simulink model "RobotX_ss_acousticsSKIP_dock_odoa_ta_1021"  (R2014a)
settings: Solver=FixedStepDiscrete  StartTime=0.0  StopTime=inf  FixedStep=.25  RelTol=1e-3
undefined symbols (not defined in the file): Com1, Com2, Com3, Com4, DiscIntNeverNeededParam, standard
libraries: xpcseriallib x42, simulink x8, slrtlib x8, speedgoatlib x2, speedgoatlib_IO102 x1
(part 5 of 19)

== matlab function RobotX_ss_acousticsSKIP_dock_odoa_ta_1021/Main FSM/ODOA/SLAM1/Models for prediction/Model10/Dynamic Model ==
  data: F_surge input; F_sway input; Torque input; u input; surgeAccel output; v input; psi input; swayAccel output; yawAccel output
function [surgeAccel, swayAccel, yawAccel] = ...
    WAM_V_3DOF(F_surge, F_sway, Torque, u, v, psi)
%Written by Anderson Lebbad on August 12, 2014
%Last Edited:

%This function was heavily based off of Ariel Qu's Vel3DOF_IvanV1. It was
%rewritten for real-time use.

%This function will produce the transient output surge velocity of a
%linearized model of the USV. It is assumed that the vehicle is equivalent
%to two cylinders in the water.

%%%%%DEFINED VARIABLE%%%%%%
%
%   Xext = Thrust from motors
%   Next = Moment from motor
%   m = Mass of vehicle
%   Xudot = Added mass in surge direction
%   Yvdot = Added mass in sway direction
%   Nrdot = Added mass from yaw
%   xg = offset from center of gravity
%   rho = density of seawater
%   S = wetted surface area
%   R = Reynolds number
%   Cd = Coefficient of drag
%   Cdc = Coefficient of drag for sway
%   nu = Kinematic viscosity
%   L = Length overall
%   T = draft
%   B = beam
%   SA = Surface area of cylinder experiencing sway
%   Iz = moment of inertia about Z axis
%
%%%%%%

% Force/Mometns from thrusters & control surfaces...

tau = [F_surge; F_sway; Torque];

% Calculate yaw rate
persistent lastHeading
if isempty(lastHeading)
    lastHeading = psi;
end
%Sample time
ts = .1;

r = (psi - lastHeading)/ts;

% Velocity & Angular velocity vectors
vel = [u; v; 0];
omega = [0; 0; r];

%define variables
m = 145.7;         % Total mass [kg] - reduced from 102
rho = 1025.9;   % density of seawater [kg/m^3]
L = 3.91*0.85;  % Length on the waterline [m]
B = 0.426;       % Demihull beam [m]
T = B*0.2;        % Draft of the demihull [m]
p_bar = 1.0; % sidehull separation - from centerplane vessel to centerplane demihull
Iz = 262.181;    % Mass moment of inertia about z-axis [kg*m^2]
xg = 0;         % Body-Fixed coordinate system taken to be center of gravity
yg = 0;         % Symmetrical Vessel
Cd = 1.1;       % Drag coefficient for a lateral cylinder
LCG = 1.485;        % Need to know where LCG wrt stern

% Vector location of port and starboard hulls
r_port = [-LCG; -p_bar; 0];   
r_stbd = [-LCG; p_bar; 0];

% Port and starboard hull velocities
vel_port = vel + cross(omega,r_port);
vel_stbd = vel + cross(omega,r_stbd);

u_port = vel_port(1);
u_stbd = vel_stbd(1);

% Port and starboard state vectors
state_port = vel_port + omega;
state_stbd = vel_stbd + omega;

%% Added Mass
% Estimated for each hull, then multiplied by 2 to account for both hulls
Xudot = -0.05*m;

%Using strip theory to estimate added mass coefficients
Nrdot = -(4.75/2*pi*rho*p_bar*T^4 + pi*rho*T^2*((L - LCG)^3 + LCG^3)/3);
Nvdot = - pi*rho*T^2*((L - LCG)^2 - LCG^2)/2;

Yrdot = Nvdot;
Yvdot = -rho*pi*T^2*L;

% Multiply by 2:
Xudot = 2*Xudot;
Nrdot = 2*Nrdot;
Nvdot = 2*Nvdot;
Yrdot = 2*Yrdot;
Yvdot = 2*Yvdot;

%Calculate Coefficient of Drag for Sway from 1950 SNAME approximation
Cdc= 1.1 + 0.0045*L/T - 0.1*B/T + 0.016*(B/T)^2;
SA = 2*pi/4*T*L; %projected area of pontoon for two pontoons

%% Linear Drag Terms
%Total Speed
U = sqrt(u^2+v^2);

Xu = 0;
Yv = -0.5*rho*abs(v)*2*Cdc*SA; %20 was the last working number %from SNAME 1950, x2 for two cylinders
%Nr = -0.5*pi*rho*U*T^2*L^2;
Nr = -pi*rho*U*T^2*L^2*.065;
Nv = -pi*rho*U*T^2*L*.01;
Yr = pi*rho*U*T^2*L*0.2;  %from Newman approximation in Lewandowski

%% Nonlinear Drag Terms

% Drag and Moment due to drag on entire vessel - includes nonlinear and
% linear drag terms
D_port = 0.5*(0.44*u_port^3 - 0.01*u_port^2 + 19*u_port);     % Can assume that this equation also takes into account Xu - so set Xu=0
D_stbd = 0.5*(0.44*u_stbd^3 - 0.01*u_stbd^2 + 19*u_stbd);     % Can assume that this equation also takes into account Xu - so set Xu=0

tau_drag = [-(D_port + D_stbd); 0; (D_stbd - D_port)*p_bar];

Xuu = 0;

%% Maneuvering Coefficient Matrices
% Added Mass Matrix
M = [(m - Xudot)      0              0;...
    0               (m - Yvdot)     (m*xg - Yrdot);...
    0               (m*xg - Nvdot)  (Iz - Nrdot)];

%Centripetal and Added Mass Centripetal force matrices
% C_RB = [
%     0                  0                0
%     0                  0                0
%     0                  0                0
%     ];

% C_RB = [
%     0                  0                -m*(xg*r + v)
%     0                  0                -m*(yg*r - u)
%     m*(xg*r + v)       m*(yg*r - u)     0
%     ];

% C_A = -[ %negative originally
%     0                               0           0
%     0                               0           0
%     0                               0           0
%     ];

% Negating centripetal acceleration for test
C_RB = 0;
C_A = 0;

D = -[Xu  0   0;...
      0   Yv  Yr;...
      0   Nv  Nr];

% Nonlinear Drag Coefficients
D_N = -[Xuu*u   0                       0;...
        0       0                       0;...
        0       0                       0];
    
%% Calculate the port and starboard force vectors
tau_port = -(C_RB + C_A + D + D_N)*state_port;
tau_stbd = -(C_RB + C_A + D + D_N)*state_stbd;


%% Sum the force vectors
tau_tot = tau + tau_drag + tau_port + tau_stbd...
    + cross(r_port,[tau_port(1);tau_port(2);0]) + ...
    cross(r_stbd,[tau_stbd(1);tau_stbd(2);0]);

% Calculate the time derivative of the state vector

accel = M\tau_tot;

%% Separate output

surgeAccel = accel(1);
swayAccel = accel(2);
yawAccel = accel(3);

end

== matlab function RobotX_ss_acousticsSKIP_dock_odoa_ta_1021/Main FSM/ODOA/SLAM1/Models for prediction/Model13/Stbd Thruster Model ==
  data: stbdMP input; F_surge output; stbdAzimuth input; F_sway output; Torque output
function [F_surge,F_sway,Torque]  = StarBoardThruster(stbdMP,stbdAzimuth)
%Approximation for Starboard Force and Moment with the input motor power
%and azimuth angle of thruster

%Longitudinal distance from center of mass
longDist =1.007;           %m

%Axial distance from center of mass
axialDist=1.485;            %m

%% Piece-wise thrust calculation

if stbdMP <= -51.0119
    F = .9140*stbdMP + 40;
elseif stbdMP >= 26.8367
    F = 1.658*stbdMP - 41.01;
else
    F = .12987*stbdMP;
end

%% Force components
F_surge=F*cos(stbdAzimuth*pi/180);       %N
F_sway=F*sin(stbdAzimuth*pi/180);       %N

%% Torque calculation

Torque = -F_surge*longDist - F_sway*axialDist;   %N.m

end

== matlab function RobotX_ss_acousticsSKIP_dock_odoa_ta_1021/Main FSM/ODOA/SLAM1/Models for prediction/Model14/Dynamic Model ==
  data: F_surge input; F_sway input; Torque input; u input; surgeAccel output; v input; psi input; swayAccel output; yawAccel output
function [surgeAccel, swayAccel, yawAccel] = ...
    WAM_V_3DOF(F_surge, F_sway, Torque, u, v, psi)
%Written by Anderson Lebbad on August 12, 2014
%Last Edited:

%This function was heavily based off of Ariel Qu's Vel3DOF_IvanV1. It was
%rewritten for real-time use.

%This function will produce the transient output surge velocity of a
%linearized model of the USV. It is assumed that the vehicle is equivalent
%to two cylinders in the water.

%%%%%DEFINED VARIABLE%%%%%%
%
%   Xext = Thrust from motors
%   Next = Moment from motor
%   m = Mass of vehicle
%   Xudot = Added mass in surge direction
%   Yvdot = Added mass in sway direction
%   Nrdot = Added mass from yaw
%   xg = offset from center of gravity
%   rho = density of seawater
%   S = wetted surface area
%   R = Reynolds number
%   Cd = Coefficient of drag
%   Cdc = Coefficient of drag for sway
%   nu = Kinematic viscosity
%   L = Length overall
%   T = draft
%   B = beam
%   SA = Surface area of cylinder experiencing sway
%   Iz = moment of inertia about Z axis
%
%%%%%%

% Force/Mometns from thrusters & control surfaces...

tau = [F_surge; F_sway; Torque];

% Calculate yaw rate
persistent lastHeading
if isempty(lastHeading)
    lastHeading = psi;
end
%Sample time
ts = .1;

r = (psi - lastHeading)/ts;

% Velocity & Angular velocity vectors
vel = [u; v; 0];
omega = [0; 0; r];

%define variables
m = 145.7;         % Total mass [kg] - reduced from 102
rho = 1025.9;   % density of seawater [kg/m^3]
L = 3.91*0.85;  % Length on the waterline [m]
B = 0.426;       % Demihull beam [m]
T = B*0.2;        % Draft of the demihull [m]
p_bar = 1.0; % sidehull separation - from centerplane vessel to centerplane demihull
Iz = 262.181;    % Mass moment of inertia about z-axis [kg*m^2]
xg = 0;         % Body-Fixed coordinate system taken to be center of gravity
yg = 0;         % Symmetrical Vessel
Cd = 1.1;       % Drag coefficient for a lateral cylinder
LCG = 1.485;        % Need to know where LCG wrt stern

% Vector location of port and starboard hulls
r_port = [-LCG; -p_bar; 0];   
r_stbd = [-LCG; p_bar; 0];

% Port and starboard hull velocities
vel_port = vel + cross(omega,r_port);
vel_stbd = vel + cross(omega,r_stbd);

u_port = vel_port(1);
u_stbd = vel_stbd(1);

% Port and starboard state vectors
state_port = vel_port + omega;
state_stbd = vel_stbd + omega;

%% Added Mass
% Estimated for each hull, then multiplied by 2 to account for both hulls
Xudot = -0.05*m;

%Using strip theory to estimate added mass coefficients
Nrdot = -(4.75/2*pi*rho*p_bar*T^4 + pi*rho*T^2*((L - LCG)^3 + LCG^3)/3);
Nvdot = - pi*rho*T^2*((L - LCG)^2 - LCG^2)/2;

Yrdot = Nvdot;
Yvdot = -rho*pi*T^2*L;

% Multiply by 2:
Xudot = 2*Xudot;
Nrdot = 2*Nrdot;
Nvdot = 2*Nvdot;
Yrdot = 2*Yrdot;
Yvdot = 2*Yvdot;

%Calculate Coefficient of Drag for Sway from 1950 SNAME approximation
Cdc= 1.1 + 0.0045*L/T - 0.1*B/T + 0.016*(B/T)^2;
SA = 2*pi/4*T*L; %projected area of pontoon for two pontoons

%% Linear Drag Terms
%Total Speed
U = sqrt(u^2+v^2);

Xu = 0;
Yv = -0.5*rho*abs(v)*2*Cdc*SA; %20 was the last working number %from SNAME 1950, x2 for two cylinders
%Nr = -0.5*pi*rho*U*T^2*L^2;
Nr = -pi*rho*U*T^2*L^2*.065;
Nv = -pi*rho*U*T^2*L*.01;
Yr = pi*rho*U*T^2*L*0.2;  %from Newman approximation in Lewandowski

%% Nonlinear Drag Terms

% Drag and Moment due to drag on entire vessel - includes nonlinear and
% linear drag terms
D_port = 0.5*(0.44*u_port^3 - 0.01*u_port^2 + 19*u_port);     % Can assume that this equation also takes into account Xu - so set Xu=0
D_stbd = 0.5*(0.44*u_stbd^3 - 0.01*u_stbd^2 + 19*u_stbd);     % Can assume that this equation also takes into account Xu - so set Xu=0

tau_drag = [-(D_port + D_stbd); 0; (D_stbd - D_port)*p_bar];

Xuu = 0;

%% Maneuvering Coefficient Matrices
% Added Mass Matrix
M = [(m - Xudot)      0              0;...
    0               (m - Yvdot)     (m*xg - Yrdot);...
    0               (m*xg - Nvdot)  (Iz - Nrdot)];

%Centripetal and Added Mass Centripetal force matrices
% C_RB = [
%     0                  0                0
%     0                  0                0
%     0                  0                0
%     ];

% C_RB = [
%     0                  0                -m*(xg*r + v)
%     0                  0                -m*(yg*r - u)
%     m*(xg*r + v)       m*(yg*r - u)     0
%     ];

% C_A = -[ %negative originally
%     0                               0           0
%     0                               0           0
%     0                               0           0
%     ];

% Negating centripetal acceleration for test
C_RB = 0;
C_A = 0;

D = -[Xu  0   0;...
      0   Yv  Yr;...
      0   Nv  Nr];

% Nonlinear Drag Coefficients
D_N = -[Xuu*u   0                       0;...
        0       0                       0;...
        0       0                       0];
    
%% Calculate the port and starboard force vectors
tau_port = -(C_RB + C_A + D + D_N)*state_port;
tau_stbd = -(C_RB + C_A + D + D_N)*state_stbd;


%% Sum the force vectors
tau_tot = tau + tau_drag + tau_port + tau_stbd...
    + cross(r_port,[tau_port(1);tau_port(2);0]) + ...
    cross(r_stbd,[tau_stbd(1);tau_stbd(2);0]);

% Calculate the time derivative of the state vector

accel = M\tau_tot;

%% Separate output

surgeAccel = accel(1);
swayAccel = accel(2);
yawAccel = accel(3);

end

== matlab function RobotX_ss_acousticsSKIP_dock_odoa_ta_1021/Main FSM/ODOA/SLAM1/Models for prediction/Model17/Stbd Thruster Model ==
  data: stbdMP input; F_surge output; stbdAzimuth input; F_sway output; Torque output
function [F_surge,F_sway,Torque]  = StarBoardThruster(stbdMP,stbdAzimuth)
%Approximation for Starboard Force and Moment with the input motor power
%and azimuth angle of thruster

%Longitudinal distance from center of mass
longDist =1.007;           %m

%Axial distance from center of mass
axialDist=1.485;            %m

%% Piece-wise thrust calculation

if stbdMP <= -51.0119
    F = .9140*stbdMP + 40;
elseif stbdMP >= 26.8367
    F = 1.658*stbdMP - 41.01;
else
    F = .12987*stbdMP;
end

%% Force components
F_surge=F*cos(stbdAzimuth*pi/180);       %N
F_sway=F*sin(stbdAzimuth*pi/180);       %N

%% Torque calculation

Torque = -F_surge*longDist - F_sway*axialDist;   %N.m

end

== matlab function RobotX_ss_acousticsSKIP_dock_odoa_ta_1021/Main FSM/ODOA/SLAM1/Models for prediction/Model18/Dynamic Model ==
  data: F_surge input; F_sway input; Torque input; u input; surgeAccel output; v input; psi input; swayAccel output; yawAccel output
function [surgeAccel, swayAccel, yawAccel] = ...
    WAM_V_3DOF(F_surge, F_sway, Torque, u, v, psi)
%Written by Anderson Lebbad on August 12, 2014
%Last Edited:

%This function was heavily based off of Ariel Qu's Vel3DOF_IvanV1. It was
%rewritten for real-time use.

%This function will produce the transient output surge velocity of a
%linearized model of the USV. It is assumed that the vehicle is equivalent
%to two cylinders in the water.

%%%%%DEFINED VARIABLE%%%%%%
%
%   Xext = Thrust from motors
%   Next = Moment from motor
%   m = Mass of vehicle
%   Xudot = Added mass in surge direction
%   Yvdot = Added mass in sway direction
%   Nrdot = Added mass from yaw
%   xg = offset from center of gravity
%   rho = density of seawater
%   S = wetted surface area
%   R = Reynolds number
%   Cd = Coefficient of drag
%   Cdc = Coefficient of drag for sway
%   nu = Kinematic viscosity
%   L = Length overall
%   T = draft
%   B = beam
%   SA = Surface area of cylinder experiencing sway
%   Iz = moment of inertia about Z axis
%
%%%%%%

% Force/Mometns from thrusters & control surfaces...

tau = [F_surge; F_sway; Torque];

% Calculate yaw rate
persistent lastHeading
if isempty(lastHeading)
    lastHeading = psi;
end
%Sample time
ts = .1;

r = (psi - lastHeading)/ts;

% Velocity & Angular velocity vectors
vel = [u; v; 0];
omega = [0; 0; r];

%define variables
m = 145.7;         % Total mass [kg] - reduced from 102
rho = 1025.9;   % density of seawater [kg/m^3]
L = 3.91*0.85;  % Length on the waterline [m]
B = 0.426;       % Demihull beam [m]
T = B*0.2;        % Draft of the demihull [m]
p_bar = 1.0; % sidehull separation - from centerplane vessel to centerplane demihull
Iz = 262.181;    % Mass moment of inertia about z-axis [kg*m^2]
xg = 0;         % Body-Fixed coordinate system taken to be center of gravity
yg = 0;         % Symmetrical Vessel
Cd = 1.1;       % Drag coefficient for a lateral cylinder
LCG = 1.485;        % Need to know where LCG wrt stern

% Vector location of port and starboard hulls
r_port = [-LCG; -p_bar; 0];   
r_stbd = [-LCG; p_bar; 0];

% Port and starboard hull velocities
vel_port = vel + cross(omega,r_port);
vel_stbd = vel + cross(omega,r_stbd);

u_port = vel_port(1);
u_stbd = vel_stbd(1);

% Port and starboard state vectors
state_port = vel_port + omega;
state_stbd = vel_stbd + omega;

%% Added Mass
% Estimated for each hull, then multiplied by 2 to account for both hulls
Xudot = -0.05*m;

%Using strip theory to estimate added mass coefficients
Nrdot = -(4.75/2*pi*rho*p_bar*T^4 + pi*rho*T^2*((L - LCG)^3 + LCG^3)/3);
Nvdot = - pi*rho*T^2*((L - LCG)^2 - LCG^2)/2;

Yrdot = Nvdot;
Yvdot = -rho*pi*T^2*L;

% Multiply by 2:
Xudot = 2*Xudot;
Nrdot = 2*Nrdot;
Nvdot = 2*Nvdot;
Yrdot = 2*Yrdot;
Yvdot = 2*Yvdot;

%Calculate Coefficient of Drag for Sway from 1950 SNAME approximation
Cdc= 1.1 + 0.0045*L/T - 0.1*B/T + 0.016*(B/T)^2;
SA = 2*pi/4*T*L; %projected area of pontoon for two pontoons

%% Linear Drag Terms
%Total Speed
U = sqrt(u^2+v^2);

Xu = 0;
Yv = -0.5*rho*abs(v)*2*Cdc*SA; %20 was the last working number %from SNAME 1950, x2 for two cylinders
%Nr = -0.5*pi*rho*U*T^2*L^2;
Nr = -pi*rho*U*T^2*L^2*.065;
Nv = -pi*rho*U*T^2*L*.01;
Yr = pi*rho*U*T^2*L*0.2;  %from Newman approximation in Lewandowski

%% Nonlinear Drag Terms

% Drag and Moment due to drag on entire vessel - includes nonlinear and
% linear drag terms
D_port = 0.5*(0.44*u_port^3 - 0.01*u_port^2 + 19*u_port);     % Can assume that this equation also takes into account Xu - so set Xu=0
D_stbd = 0.5*(0.44*u_stbd^3 - 0.01*u_stbd^2 + 19*u_stbd);     % Can assume that this equation also takes into account Xu - so set Xu=0

tau_drag = [-(D_port + D_stbd); 0; (D_stbd - D_port)*p_bar];

Xuu = 0;

%% Maneuvering Coefficient Matrices
% Added Mass Matrix
M = [(m - Xudot)      0              0;...
    0               (m - Yvdot)     (m*xg - Yrdot);...
    0               (m*xg - Nvdot)  (Iz - Nrdot)];

%Centripetal and Added Mass Centripetal force matrices
% C_RB = [
%     0                  0                0
%     0                  0                0
%     0                  0                0
%     ];

% C_RB = [
%     0                  0                -m*(xg*r + v)
%     0                  0                -m*(yg*r - u)
%     m*(xg*r + v)       m*(yg*r - u)     0
%     ];

% C_A = -[ %negative originally
%     0                               0           0
%     0                               0           0
%     0                               0           0
%     ];

% Negating centripetal acceleration for test
C_RB = 0;
C_A = 0;

D = -[Xu  0   0;...
      0   Yv  Yr;...
      0   Nv  Nr];

% Nonlinear Drag Coefficients
D_N = -[Xuu*u   0                       0;...
        0       0                       0;...
        0       0                       0];
    
%% Calculate the port and starboard force vectors
tau_port = -(C_RB + C_A + D + D_N)*state_port;
tau_stbd = -(C_RB + C_A + D + D_N)*state_stbd;


%% Sum the force vectors
tau_tot = tau + tau_drag + tau_port + tau_stbd...
    + cross(r_port,[tau_port(1);tau_port(2);0]) + ...
    cross(r_stbd,[tau_stbd(1);tau_stbd(2);0]);

% Calculate the time derivative of the state vector

accel = M\tau_tot;

%% Separate output

surgeAccel = accel(1);
swayAccel = accel(2);
yawAccel = accel(3);

end

== matlab function RobotX_ss_acousticsSKIP_dock_odoa_ta_1021/Main FSM/ODOA/SLAM1/Models for prediction/Model20/Stbd Thruster Model ==
  data: stbdMP input; F_surge output; stbdAzimuth input; F_sway output; Torque output
function [F_surge,F_sway,Torque]  = StarBoardThruster(stbdMP,stbdAzimuth)
%Approximation for Starboard Force and Moment with the input motor power
%and azimuth angle of thruster

%Longitudinal distance from center of mass
longDist =1.007;           %m

%Axial distance from center of mass
axialDist=1.485;            %m

%% Piece-wise thrust calculation

if stbdMP <= -51.0119
    F = .9140*stbdMP + 40;
elseif stbdMP >= 26.8367
    F = 1.658*stbdMP - 41.01;
else
    F = .12987*stbdMP;
end

%% Force components
F_surge=F*cos(stbdAzimuth*pi/180);       %N
F_sway=F*sin(stbdAzimuth*pi/180);       %N

%% Torque calculation

Torque = -F_surge*longDist - F_sway*axialDist;   %N.m

end

== matlab function RobotX_ss_acousticsSKIP_dock_odoa_ta_1021/Main FSM/ODOA/SLAM1/Models for prediction/Model21/Dynamic Model ==
  data: F_surge input; F_sway input; Torque input; u input; surgeAccel output; v input; psi input; swayAccel output; yawAccel output
function [surgeAccel, swayAccel, yawAccel] = ...
    WAM_V_3DOF(F_surge, F_sway, Torque, u, v, psi)
%Written by Anderson Lebbad on August 12, 2014
%Last Edited:

%This function was heavily based off of Ariel Qu's Vel3DOF_IvanV1. It was
%rewritten for real-time use.

%This function will produce the transient output surge velocity of a
%linearized model of the USV. It is assumed that the vehicle is equivalent
%to two cylinders in the water.

%%%%%DEFINED VARIABLE%%%%%%
%
%   Xext = Thrust from motors
%   Next = Moment from motor
%   m = Mass of vehicle
%   Xudot = Added mass in surge direction
%   Yvdot = Added mass in sway direction
%   Nrdot = Added mass from yaw
%   xg = offset from center of gravity
%   rho = density of seawater
%   S = wetted surface area
%   R = Reynolds number
%   Cd = Coefficient of drag
%   Cdc = Coefficient of drag for sway
%   nu = Kinematic viscosity
%   L = Length overall
%   T = draft
%   B = beam
%   SA = Surface area of cylinder experiencing sway
%   Iz = moment of inertia about Z axis
%
%%%%%%

% Force/Mometns from thrusters & control surfaces...

tau = [F_surge; F_sway; Torque];

% Calculate yaw rate
persistent lastHeading
if isempty(lastHeading)
    lastHeading = psi;
end
%Sample time
ts = .1;

r = (psi - lastHeading)/ts;

% Velocity & Angular velocity vectors
vel = [u; v; 0];
omega = [0; 0; r];

%define variables
m = 145.7;         % Total mass [kg] - reduced from 102
rho = 1025.9;   % density of seawater [kg/m^3]
L = 3.91*0.85;  % Length on the waterline [m]
B = 0.426;       % Demihull beam [m]
T = B*0.2;        % Draft of the demihull [m]
p_bar = 1.0; % sidehull separation - from centerplane vessel to centerplane demihull
Iz = 262.181;    % Mass moment of inertia about z-axis [kg*m^2]
xg = 0;         % Body-Fixed coordinate system taken to be center of gravity
yg = 0;         % Symmetrical Vessel
Cd = 1.1;       % Drag coefficient for a lateral cylinder
LCG = 1.485;        % Need to know where LCG wrt stern

% Vector location of port and starboard hulls
r_port = [-LCG; -p_bar; 0];   
r_stbd = [-LCG; p_bar; 0];

% Port and starboard hull velocities
vel_port = vel + cross(omega,r_port);
vel_stbd = vel + cross(omega,r_stbd);

u_port = vel_port(1);
u_stbd = vel_stbd(1);

% Port and starboard state vectors
state_port = vel_port + omega;
state_stbd = vel_stbd + omega;

%% Added Mass
% Estimated for each hull, then multiplied by 2 to account for both hulls
Xudot = -0.05*m;

%Using strip theory to estimate added mass coefficients
Nrdot = -(4.75/2*pi*rho*p_bar*T^4 + pi*rho*T^2*((L - LCG)^3 + LCG^3)/3);
Nvdot = - pi*rho*T^2*((L - LCG)^2 - LCG^2)/2;

Yrdot = Nvdot;
Yvdot = -rho*pi*T^2*L;

% Multiply by 2:
Xudot = 2*Xudot;
Nrdot = 2*Nrdot;
Nvdot = 2*Nvdot;
Yrdot = 2*Yrdot;
Yvdot = 2*Yvdot;

%Calculate Coefficient of Drag for Sway from 1950 SNAME approximation
Cdc= 1.1 + 0.0045*L/T - 0.1*B/T + 0.016*(B/T)^2;
SA = 2*pi/4*T*L; %projected area of pontoon for two pontoons

%% Linear Drag Terms
%Total Speed
U = sqrt(u^2+v^2);

Xu = 0;
Yv = -0.5*rho*abs(v)*2*Cdc*SA; %20 was the last working number %from SNAME 1950, x2 for two cylinders
%Nr = -0.5*pi*rho*U*T^2*L^2;
Nr = -pi*rho*U*T^2*L^2*.065;
Nv = -pi*rho*U*T^2*L*.01;
Yr = pi*rho*U*T^2*L*0.2;  %from Newman approximation in Lewandowski

%% Nonlinear Drag Terms

% Drag and Moment due to drag on entire vessel - includes nonlinear and
% linear drag terms
D_port = 0.5*(0.44*u_port^3 - 0.01*u_port^2 + 19*u_port);     % Can assume that this equation also takes into account Xu - so set Xu=0
D_stbd = 0.5*(0.44*u_stbd^3 - 0.01*u_stbd^2 + 19*u_stbd);     % Can assume that this equation also takes into account Xu - so set Xu=0

tau_drag = [-(D_port + D_stbd); 0; (D_stbd - D_port)*p_bar];

Xuu = 0;

%% Maneuvering Coefficient Matrices
% Added Mass Matrix
M = [(m - Xudot)      0              0;...
    0               (m - Yvdot)     (m*xg - Yrdot);...
    0               (m*xg - Nvdot)  (Iz - Nrdot)];

%Centripetal and Added Mass Centripetal force matrices
% C_RB = [
%     0                  0                0
%     0                  0                0
%     0                  0                0
%     ];

% C_RB = [
%     0                  0                -m*(xg*r + v)
%     0                  0                -m*(yg*r - u)
%     m*(xg*r + v)       m*(yg*r - u)     0
%     ];

% C_A = -[ %negative originally
%     0                               0           0
%     0                               0           0
%     0                               0           0
%     ];

% Negating centripetal acceleration for test
C_RB = 0;
C_A = 0;

D = -[Xu  0   0;...
      0   Yv  Yr;...
      0   Nv  Nr];

% Nonlinear Drag Coefficients
D_N = -[Xuu*u   0                       0;...
        0       0                       0;...
        0       0                       0];
    
%% Calculate the port and starboard force vectors
tau_port = -(C_RB + C_A + D + D_N)*state_port;
tau_stbd = -(C_RB + C_A + D + D_N)*state_stbd;


%% Sum the force vectors
tau_tot = tau + tau_drag + tau_port + tau_stbd...
    + cross(r_port,[tau_port(1);tau_port(2);0]) + ...
    cross(r_stbd,[tau_stbd(1);tau_stbd(2);0]);

% Calculate the time derivative of the state vector

accel = M\tau_tot;

%% Separate output

surgeAccel = accel(1);
swayAccel = accel(2);
yawAccel = accel(3);

end

== matlab function RobotX_ss_acousticsSKIP_dock_odoa_ta_1021/Main FSM/ODOA/SLAM1/Models for prediction/Model24/Stbd Thruster Model ==
  data: stbdMP input; F_surge output; stbdAzimuth input; F_sway output; Torque output
function [F_surge,F_sway,Torque]  = StarBoardThruster(stbdMP,stbdAzimuth)
%Approximation for Starboard Force and Moment with the input motor power
%and azimuth angle of thruster

%Longitudinal distance from center of mass
longDist =1.007;           %m

%Axial distance from center of mass
axialDist=1.485;            %m

%% Piece-wise thrust calculation

if stbdMP <= -51.0119
    F = .9140*stbdMP + 40;
elseif stbdMP >= 26.8367
    F = 1.658*stbdMP - 41.01;
else
    F = .12987*stbdMP;
end

%% Force components
F_surge=F*cos(stbdAzimuth*pi/180);       %N
F_sway=F*sin(stbdAzimuth*pi/180);       %N

%% Torque calculation

Torque = -F_surge*longDist - F_sway*axialDist;   %N.m

end

== matlab function RobotX_ss_acousticsSKIP_dock_odoa_ta_1021/Main FSM/ODOA/SLAM1/Models for prediction/Model25/Dynamic Model ==
  data: F_surge input; F_sway input; Torque input; u input; surgeAccel output; v input; psi input; swayAccel output; yawAccel output
function [surgeAccel, swayAccel, yawAccel] = ...
    WAM_V_3DOF(F_surge, F_sway, Torque, u, v, psi)
%Written by Anderson Lebbad on August 12, 2014
%Last Edited:

%This function was heavily based off of Ariel Qu's Vel3DOF_IvanV1. It was
%rewritten for real-time use.

%This function will produce the transient output surge velocity of a
%linearized model of the USV. It is assumed that the vehicle is equivalent
%to two cylinders in the water.

%%%%%DEFINED VARIABLE%%%%%%
%
%   Xext = Thrust from motors
%   Next = Moment from motor
%   m = Mass of vehicle
%   Xudot = Added mass in surge direction
%   Yvdot = Added mass in sway direction
%   Nrdot = Added mass from yaw
%   xg = offset from center of gravity
%   rho = density of seawater
%   S = wetted surface area
%   R = Reynolds number
%   Cd = Coefficient of drag
%   Cdc = Coefficient of drag for sway
%   nu = Kinematic viscosity
%   L = Length overall
%   T = draft
%   B = beam
%   SA = Surface area of cylinder experiencing sway
%   Iz = moment of inertia about Z axis
%
%%%%%%

% Force/Mometns from thrusters & control surfaces...

tau = [F_surge; F_sway; Torque];

% Calculate yaw rate
persistent lastHeading
if isempty(lastHeading)
    lastHeading = psi;
end
%Sample time
ts = .1;

r = (psi - lastHeading)/ts;

% Velocity & Angular velocity vectors
vel = [u; v; 0];
omega = [0; 0; r];

%define variables
m = 145.7;         % Total mass [kg] - reduced from 102
rho = 1025.9;   % density of seawater [kg/m^3]
L = 3.91*0.85;  % Length on the waterline [m]
B = 0.426;       % Demihull beam [m]
T = B*0.2;        % Draft of the demihull [m]
p_bar = 1.0; % sidehull separation - from centerplane vessel to centerplane demihull
Iz = 262.181;    % Mass moment of inertia about z-axis [kg*m^2]
xg = 0;         % Body-Fixed coordinate system taken to be center of gravity
yg = 0;         % Symmetrical Vessel
Cd = 1.1;       % Drag coefficient for a lateral cylinder
LCG = 1.485;        % Need to know where LCG wrt stern

% Vector location of port and starboard hulls
r_port = [-LCG; -p_bar; 0];   
r_stbd = [-LCG; p_bar; 0];

% Port and starboard hull velocities
vel_port = vel + cross(omega,r_port);
vel_stbd = vel + cross(omega,r_stbd);

u_port = vel_port(1);
u_stbd = vel_stbd(1);

% Port and starboard state vectors
state_port = vel_port + omega;
state_stbd = vel_stbd + omega;

%% Added Mass
% Estimated for each hull, then multiplied by 2 to account for both hulls
Xudot = -0.05*m;

%Using strip theory to estimate added mass coefficients
Nrdot = -(4.75/2*pi*rho*p_bar*T^4 + pi*rho*T^2*((L - LCG)^3 + LCG^3)/3);
Nvdot = - pi*rho*T^2*((L - LCG)^2 - LCG^2)/2;

Yrdot = Nvdot;
Yvdot = -rho*pi*T^2*L;

% Multiply by 2:
Xudot = 2*Xudot;
Nrdot = 2*Nrdot;
Nvdot = 2*Nvdot;
Yrdot = 2*Yrdot;
Yvdot = 2*Yvdot;

%Calculate Coefficient of Drag for Sway from 1950 SNAME approximation
Cdc= 1.1 + 0.0045*L/T - 0.1*B/T + 0.016*(B/T)^2;
SA = 2*pi/4*T*L; %projected area of pontoon for two pontoons

%% Linear Drag Terms
%Total Speed
U = sqrt(u^2+v^2);

Xu = 0;
Yv = -0.5*rho*abs(v)*2*Cdc*SA; %20 was the last working number %from SNAME 1950, x2 for two cylinders
%Nr = -0.5*pi*rho*U*T^2*L^2;
Nr = -pi*rho*U*T^2*L^2*.065;
Nv = -pi*rho*U*T^2*L*.01;
Yr = pi*rho*U*T^2*L*0.2;  %from Newman approximation in Lewandowski

%% Nonlinear Drag Terms

% Drag and Moment due to drag on entire vessel - includes nonlinear and
% linear drag terms
D_port = 0.5*(0.44*u_port^3 - 0.01*u_port^2 + 19*u_port);     % Can assume that this equation also takes into account Xu - so set Xu=0
D_stbd = 0.5*(0.44*u_stbd^3 - 0.01*u_stbd^2 + 19*u_stbd);     % Can assume that this equation also takes into account Xu - so set Xu=0

tau_drag = [-(D_port + D_stbd); 0; (D_stbd - D_port)*p_bar];

Xuu = 0;

%% Maneuvering Coefficient Matrices
% Added Mass Matrix
M = [(m - Xudot)      0              0;...
    0               (m - Yvdot)     (m*xg - Yrdot);...
    0               (m*xg - Nvdot)  (Iz - Nrdot)];

%Centripetal and Added Mass Centripetal force matrices
% C_RB = [
%     0                  0                0
%     0                  0                0
%     0                  0                0
%     ];

% C_RB = [
%     0                  0                -m*(xg*r + v)
%     0                  0                -m*(yg*r - u)
%     m*(xg*r + v)       m*(yg*r - u)     0
%     ];

% C_A = -[ %negative originally
%     0                               0           0
%     0                               0           0
%     0                               0           0
%     ];

% Negating centripetal acceleration for test
C_RB = 0;
C_A = 0;

D = -[Xu  0   0;...
      0   Yv  Yr;...
      0   Nv  Nr];

% Nonlinear Drag Coefficients
D_N = -[Xuu*u   0                       0;...
        0       0                       0;...
        0       0                       0];
    
%% Calculate the port and starboard force vectors
tau_port = -(C_RB + C_A + D + D_N)*state_port;
tau_stbd = -(C_RB + C_A + D + D_N)*state_stbd;


%% Sum the force vectors
tau_tot = tau + tau_drag + tau_port + tau_stbd...
    + cross(r_port,[tau_port(1);tau_port(2);0]) + ...
    cross(r_stbd,[tau_stbd(1);tau_stbd(2);0]);

% Calculate the time derivative of the state vector

accel = M\tau_tot;

%% Separate output

surgeAccel = accel(1);
swayAccel = accel(2);
yawAccel = accel(3);

end

== matlab function RobotX_ss_acousticsSKIP_dock_odoa_ta_1021/Main FSM/ODOA/SLAM1/Models for prediction/Model28/Stbd Thruster Model ==
  data: stbdMP input; F_surge output; stbdAzimuth input; F_sway output; Torque output
function [F_surge,F_sway,Torque]  = StarBoardThruster(stbdMP,stbdAzimuth)
%Approximation for Starboard Force and Moment with the input motor power
%and azimuth angle of thruster

%Longitudinal distance from center of mass
longDist =1.007;           %m

%Axial distance from center of mass
axialDist=1.485;            %m

%% Piece-wise thrust calculation

if stbdMP <= -51.0119
    F = .9140*stbdMP + 40;
elseif stbdMP >= 26.8367
    F = 1.658*stbdMP - 41.01;
else
    F = .12987*stbdMP;
end

%% Force components
F_surge=F*cos(stbdAzimuth*pi/180);       %N
F_sway=F*sin(stbdAzimuth*pi/180);       %N

%% Torque calculation

Torque = -F_surge*longDist - F_sway*axialDist;   %N.m

end

== matlab function RobotX_ss_acousticsSKIP_dock_odoa_ta_1021/Main FSM/ODOA/SLAM1/Models for prediction/Model29/Dynamic Model ==
  data: F_surge input; F_sway input; Torque input; u input; surgeAccel output; v input; psi input; swayAccel output; yawAccel output
function [surgeAccel, swayAccel, yawAccel] = ...
    WAM_V_3DOF(F_surge, F_sway, Torque, u, v, psi)
%Written by Anderson Lebbad on August 12, 2014
%Last Edited:

%This function was heavily based off of Ariel Qu's Vel3DOF_IvanV1. It was
%rewritten for real-time use.

%This function will produce the transient output surge velocity of a
%linearized model of the USV. It is assumed that the vehicle is equivalent
%to two cylinders in the water.

%%%%%DEFINED VARIABLE%%%%%%
%
%   Xext = Thrust from motors
%   Next = Moment from motor
%   m = Mass of vehicle
%   Xudot = Added mass in surge direction
%   Yvdot = Added mass in sway direction
%   Nrdot = Added mass from yaw
%   xg = offset from center of gravity
%   rho = density of seawater
%   S = wetted surface area
%   R = Reynolds number
%   Cd = Coefficient of drag
%   Cdc = Coefficient of drag for sway
%   nu = Kinematic viscosity
%   L = Length overall
%   T = draft
%   B = beam
%   SA = Surface area of cylinder experiencing sway
%   Iz = moment of inertia about Z axis
%
%%%%%%

% Force/Mometns from thrusters & control surfaces...

tau = [F_surge; F_sway; Torque];

% Calculate yaw rate
persistent lastHeading
if isempty(lastHeading)
    lastHeading = psi;
end
%Sample time
ts = .1;

r = (psi - lastHeading)/ts;

% Velocity & Angular velocity vectors
vel = [u; v; 0];
omega = [0; 0; r];

%define variables
m = 145.7;         % Total mass [kg] - reduced from 102
rho = 1025.9;   % density of seawater [kg/m^3]
L = 3.91*0.85;  % Length on the waterline [m]
B = 0.426;       % Demihull beam [m]
T = B*0.2;        % Draft of the demihull [m]
p_bar = 1.0; % sidehull separation - from centerplane vessel to centerplane demihull
Iz = 262.181;    % Mass moment of inertia about z-axis [kg*m^2]
xg = 0;         % Body-Fixed coordinate system taken to be center of gravity
yg = 0;         % Symmetrical Vessel
Cd = 1.1;       % Drag coefficient for a lateral cylinder
LCG = 1.485;        % Need to know where LCG wrt stern

% Vector location of port and starboard hulls
r_port = [-LCG; -p_bar; 0];   
r_stbd = [-LCG; p_bar; 0];

% Port and starboard hull velocities
vel_port = vel + cross(omega,r_port);
vel_stbd = vel + cross(omega,r_stbd);

u_port = vel_port(1);
u_stbd = vel_stbd(1);

% Port and starboard state vectors
state_port = vel_port + omega;
state_stbd = vel_stbd + omega;

%% Added Mass
% Estimated for each hull, then multiplied by 2 to account for both hulls
Xudot = -0.05*m;

%Using strip theory to estimate added mass coefficients
Nrdot = -(4.75/2*pi*rho*p_bar*T^4 + pi*rho*T^2*((L - LCG)^3 + LCG^3)/3);
Nvdot = - pi*rho*T^2*((L - LCG)^2 - LCG^2)/2;

Yrdot = Nvdot;
Yvdot = -rho*pi*T^2*L;

% Multiply by 2:
Xudot = 2*Xudot;
Nrdot = 2*Nrdot;
Nvdot = 2*Nvdot;
Yrdot = 2*Yrdot;
Yvdot = 2*Yvdot;

%Calculate Coefficient of Drag for Sway from 1950 SNAME approximation
Cdc= 1.1 + 0.0045*L/T - 0.1*B/T + 0.016*(B/T)^2;
SA = 2*pi/4*T*L; %projected area of pontoon for two pontoons

%% Linear Drag Terms
%Total Speed
U = sqrt(u^2+v^2);

Xu = 0;
Yv = -0.5*rho*abs(v)*2*Cdc*SA; %20 was the last working number %from SNAME 1950, x2 for two cylinders
%Nr = -0.5*pi*rho*U*T^2*L^2;
Nr = -pi*rho*U*T^2*L^2*.065;
Nv = -pi*rho*U*T^2*L*.01;
Yr = pi*rho*U*T^2*L*0.2;  %from Newman approximation in Lewandowski

%% Nonlinear Drag Terms

% Drag and Moment due to drag on entire vessel - includes nonlinear and
% linear drag terms
D_port = 0.5*(0.44*u_port^3 - 0.01*u_port^2 + 19*u_port);     % Can assume that this equation also takes into account Xu - so set Xu=0
D_stbd = 0.5*(0.44*u_stbd^3 - 0.01*u_stbd^2 + 19*u_stbd);     % Can assume that this equation also takes into account Xu - so set Xu=0

tau_drag = [-(D_port + D_stbd); 0; (D_stbd - D_port)*p_bar];

Xuu = 0;

%% Maneuvering Coefficient Matrices
% Added Mass Matrix
M = [(m - Xudot)      0              0;...
    0               (m - Yvdot)     (m*xg - Yrdot);...
    0               (m*xg - Nvdot)  (Iz - Nrdot)];

%Centripetal and Added Mass Centripetal force matrices
% C_RB = [
%     0                  0                0
%     0                  0                0
%     0                  0                0
%     ];

% C_RB = [
%     0                  0                -m*(xg*r + v)
%     0                  0                -m*(yg*r - u)
%     m*(xg*r + v)       m*(yg*r - u)     0
%     ];

% C_A = -[ %negative originally
%     0                               0           0
%     0                               0           0
%     0                               0           0
%     ];

% Negating centripetal acceleration for test
C_RB = 0;
C_A = 0;

D = -[Xu  0   0;...
      0   Yv  Yr;...
      0   Nv  Nr];

% Nonlinear Drag Coefficients
D_N = -[Xuu*u   0                       0;...
        0       0                       0;...
        0       0                       0];
    
%% Calculate the port and starboard force vectors
tau_port = -(C_RB + C_A + D + D_N)*state_port;
tau_stbd = -(C_RB + C_A + D + D_N)*state_stbd;


%% Sum the force vectors
tau_tot = tau + tau_drag + tau_port + tau_stbd...
    + cross(r_port,[tau_port(1);tau_port(2);0]) + ...
    cross(r_stbd,[tau_stbd(1);tau_stbd(2);0]);

% Calculate the time derivative of the state vector

accel = M\tau_tot;

%% Separate output

surgeAccel = accel(1);
swayAccel = accel(2);
yawAccel = accel(3);

end

== matlab function RobotX_ss_acousticsSKIP_dock_odoa_ta_1021/Main FSM/ODOA/SLAM1/Models for prediction/Model31/Stbd Thruster Model ==
  data: stbdMP input; F_surge output; stbdAzimuth input; F_sway output; Torque output
function [F_surge,F_sway,Torque]  = StarBoardThruster(stbdMP,stbdAzimuth)
%Approximation for Starboard Force and Moment with the input motor power
%and azimuth angle of thruster

%Longitudinal distance from center of mass
longDist =1.007;           %m

%Axial distance from center of mass
axialDist=1.485;            %m

%% Piece-wise thrust calculation

if stbdMP <= -51.0119
    F = .9140*stbdMP + 40;
elseif stbdMP >= 26.8367
    F = 1.658*stbdMP - 41.01;
else
    F = .12987*stbdMP;
end

%% Force components
F_surge=F*cos(stbdAzimuth*pi/180);       %N
F_sway=F*sin(stbdAzimuth*pi/180);       %N

%% Torque calculation

Torque = -F_surge*longDist - F_sway*axialDist;   %N.m

end

== matlab function RobotX_ss_acousticsSKIP_dock_odoa_ta_1021/Main FSM/ODOA/SLAM1/Models for prediction/Model32/Dynamic Model ==
  data: F_surge input; F_sway input; Torque input; u input; surgeAccel output; v input; psi input; swayAccel output; yawAccel output
function [surgeAccel, swayAccel, yawAccel] = ...
    WAM_V_3DOF(F_surge, F_sway, Torque, u, v, psi)
%Written by Anderson Lebbad on August 12, 2014
%Last Edited:

%This function was heavily based off of Ariel Qu's Vel3DOF_IvanV1. It was
%rewritten for real-time use.

%This function will produce the transient output surge velocity of a
%linearized model of the USV. It is assumed that the vehicle is equivalent
%to two cylinders in the water.

%%%%%DEFINED VARIABLE%%%%%%
%
%   Xext = Thrust from motors
%   Next = Moment from motor
%   m = Mass of vehicle
%   Xudot = Added mass in surge direction
%   Yvdot = Added mass in sway direction
%   Nrdot = Added mass from yaw
%   xg = offset from center of gravity
%   rho = density of seawater
%   S = wetted surface area
%   R = Reynolds number
%   Cd = Coefficient of drag
%   Cdc = Coefficient of drag for sway
%   nu = Kinematic viscosity
%   L = Length overall
%   T = draft
%   B = beam
%   SA = Surface area of cylinder experiencing sway
%   Iz = moment of inertia about Z axis
%
%%%%%%

% Force/Mometns from thrusters & control surfaces...

tau = [F_surge; F_sway; Torque];

% Calculate yaw rate
persistent lastHeading
if isempty(lastHeading)
    lastHeading = psi;
end
%Sample time
ts = .1;

r = (psi - lastHeading)/ts;

% Velocity & Angular velocity vectors
vel = [u; v; 0];
omega = [0; 0; r];

%define variables
m = 145.7;         % Total mass [kg] - reduced from 102
rho = 1025.9;   % density of seawater [kg/m^3]
L = 3.91*0.85;  % Length on the waterline [m]
B = 0.426;       % Demihull beam [m]
T = B*0.2;        % Draft of the demihull [m]
p_bar = 1.0; % sidehull separation - from centerplane vessel to centerplane demihull
Iz = 262.181;    % Mass moment of inertia about z-axis [kg*m^2]
xg = 0;         % Body-Fixed coordinate system taken to be center of gravity
yg = 0;         % Symmetrical Vessel
Cd = 1.1;       % Drag coefficient for a lateral cylinder
LCG = 1.485;        % Need to know where LCG wrt stern

% Vector location of port and starboard hulls
r_port = [-LCG; -p_bar; 0];   
r_stbd = [-LCG; p_bar; 0];

% Port and starboard hull velocities
vel_port = vel + cross(omega,r_port);
vel_stbd = vel + cross(omega,r_stbd);

u_port = vel_port(1);
u_stbd = vel_stbd(1);

% Port and starboard state vectors
state_port = vel_port + omega;
state_stbd = vel_stbd + omega;

%% Added Mass
% Estimated for each hull, then multiplied by 2 to account for both hulls
Xudot = -0.05*m;

%Using strip theory to estimate added mass coefficients
Nrdot = -(4.75/2*pi*rho*p_bar*T^4 + pi*rho*T^2*((L - LCG)^3 + LCG^3)/3);
Nvdot = - pi*rho*T^2*((L - LCG)^2 - LCG^2)/2;

Yrdot = Nvdot;
Yvdot = -rho*pi*T^2*L;

% Multiply by 2:
Xudot = 2*Xudot;
Nrdot = 2*Nrdot;
Nvdot = 2*Nvdot;
Yrdot = 2*Yrdot;
Yvdot = 2*Yvdot;

%Calculate Coefficient of Drag for Sway from 1950 SNAME approximation
Cdc= 1.1 + 0.0045*L/T - 0.1*B/T + 0.016*(B/T)^2;
SA = 2*pi/4*T*L; %projected area of pontoon for two pontoons

%% Linear Drag Terms
%Total Speed
U = sqrt(u^2+v^2);

Xu = 0;
Yv = -0.5*rho*abs(v)*2*Cdc*SA; %20 was the last working number %from SNAME 1950, x2 for two cylinders
%Nr = -0.5*pi*rho*U*T^2*L^2;
Nr = -pi*rho*U*T^2*L^2*.065;
Nv = -pi*rho*U*T^2*L*.01;
Yr = pi*rho*U*T^2*L*0.2;  %from Newman approximation in Lewandowski

%% Nonlinear Drag Terms

% Drag and Moment due to drag on entire vessel - includes nonlinear and
% linear drag terms
D_port = 0.5*(0.44*u_port^3 - 0.01*u_port^2 + 19*u_port);     % Can assume that this equation also takes into account Xu - so set Xu=0
D_stbd = 0.5*(0.44*u_stbd^3 - 0.01*u_stbd^2 + 19*u_stbd);     % Can assume that this equation also takes into account Xu - so set Xu=0

tau_drag = [-(D_port + D_stbd); 0; (D_stbd - D_port)*p_bar];

Xuu = 0;

%% Maneuvering Coefficient Matrices
% Added Mass Matrix
M = [(m - Xudot)      0              0;...
    0               (m - Yvdot)     (m*xg - Yrdot);...
    0               (m*xg - Nvdot)  (Iz - Nrdot)];

%Centripetal and Added Mass Centripetal force matrices
% C_RB = [
%     0                  0                0
%     0                  0                0
%     0                  0                0
%     ];

% C_RB = [
%     0                  0                -m*(xg*r + v)
%     0                  0                -m*(yg*r - u)
%     m*(xg*r + v)       m*(yg*r - u)     0
%     ];

% C_A = -[ %negative originally
%     0                               0           0
%     0                               0           0
%     0                               0           0
%     ];

% Negating centripetal acceleration for test
C_RB = 0;
C_A = 0;

D = -[Xu  0   0;...
      0   Yv  Yr;...
      0   Nv  Nr];

% Nonlinear Drag Coefficients
D_N = -[Xuu*u   0                       0;...
        0       0                       0;...
        0       0                       0];
    
%% Calculate the port and starboard force vectors
tau_port = -(C_RB + C_A + D + D_N)*state_port;
tau_stbd = -(C_RB + C_A + D + D_N)*state_stbd;


%% Sum the force vectors
tau_tot = tau + tau_drag + tau_port + tau_stbd...
    + cross(r_port,[tau_port(1);tau_port(2);0]) + ...
    cross(r_stbd,[tau_stbd(1);tau_stbd(2);0]);

% Calculate the time derivative of the state vector

accel = M\tau_tot;

%% Separate output

surgeAccel = accel(1);
swayAccel = accel(2);
yawAccel = accel(3);

end

== matlab function RobotX_ss_acousticsSKIP_dock_odoa_ta_1021/Main FSM/ODOA/SLAM1/Models for prediction/Model35/Stbd Thruster Model ==
  data: stbdMP input; F_surge output; stbdAzimuth input; F_sway output; Torque output
function [F_surge,F_sway,Torque]  = StarBoardThruster(stbdMP,stbdAzimuth)
%Approximation for Starboard Force and Moment with the input motor power
%and azimuth angle of thruster

%Longitudinal distance from center of mass
longDist =1.007;           %m

%Axial distance from center of mass
axialDist=1.485;            %m

%% Piece-wise thrust calculation

if stbdMP <= -51.0119
    F = .9140*stbdMP + 40;
elseif stbdMP >= 26.8367
    F = 1.658*stbdMP - 41.01;
else
    F = .12987*stbdMP;
end

%% Force components
F_surge=F*cos(stbdAzimuth*pi/180);       %N
F_sway=F*sin(stbdAzimuth*pi/180);       %N

%% Torque calculation

Torque = -F_surge*longDist - F_sway*axialDist;   %N.m

end
